simulink model "RemoteMicrogrid"  (R2025a)
settings: Solver=FixedStepAuto  StartTime=0.0  StopTime=8  FixedStep=Ts  MaxStep=1e-3  RelTol=1e-3
PreLoadFcn:
  | RemoteMicrogridInputData
undefined symbols (not defined in the file): BESS, ControlRoom, DiscIntNeverNeededParam, Grid, Load, Machine, Microgrid, MicrogridStatus, PV, relay1, T_on, Ts
libraries: ee_lib x53, fl_lib x39, eeGeneralControl x30, simulink x30, nesl_utility x26, nesl_utility_internal x19, slpidlib x7, eeTransforms x5, eeRmsMeasurement x4, eeTotalHarmonicDistorsion x4, batteryecm_lib x2, simulink_extras x2
(part 6 of 6)

== matlab function RemoteMicrogrid/Operator Control Room/Microgrid Control/Protection & Power Tracking/Overcurrent relay/Phase Protection Unit/Operating time /MATLAB Function ==
  data: plugSetting input; operatingTime output; timeSetting input; relayCharacteristic input
function operatingTime = fcn(plugSetting,timeSetting,relayCharacteristic)
   if plugSetting(1)>1 || plugSetting(2)>1 || plugSetting(3)>1  % Fault condition
    switch relayCharacteristic  % Selection of relay characteristic
        case 1                  % IEC Normal Inverse
          a=0.14;      
          b=0.02;
          c=0;
        case 2                  % IEC Very Inverse
           a=13.5;
           b=1;
           c=0;
        case 3                  % IEC Extremely Inverse
            a=80;
            b=2;
            c=0;
        case 4                  % IEC Moderately Inverse
            a=0.0515;
            b=0.02;
            c=0.114;
        case 5                  % IEEE Very Inverse
            a=19.61;
            b=2;
            c=0.491;
        case 6                  % IEEE Exteremely Inverse
            a=28.2;
            b=2;
            c=0.1217;
        otherwise               % Definite Time
            a=1;
            b=1;
            c=0;
            plugSetting=ones(3,1)*2;
    end           
         
         operatingTime=timeSetting*(a/(power(max(plugSetting),b)-1)+c);  % Calculate oeprating time of the relay  
   else
         operatingTime=inf;  % Set relay operating time to infinite if there is no fault
   end
end

== stateflow chart RemoteMicrogrid/Diesel Substation, BESS, & Microgrid Controller/Microgrid Controller/Microgrid Supervisory Control/Transition and Dispatch Control/On.Steady_State_Grid_Connected ==
  state Steady_State
    emergencyDispatch = false;
  state Resync_actions
    loadDispatch = true;
    LoadF2A = 0;
    LoadF2B = 0;
    loadReference = 0.1;
  (default) -> Steady_State
  Steady_State -> Resync_actions : after(0.2,sec)[resyncDispatch == true]
  data: LoadF2A output; LoadF2B output double; loadDispatch output boolean; loadReference output double; emergencyDispatch output boolean; resyncDispatch input boolean size=1

== stateflow chart RemoteMicrogrid/Diesel Substation, BESS, & Microgrid Controller/Microgrid Controller/Microgrid Supervisory Control/Transition and Dispatch Control/On.Resynchronization ==
  state Enable
    resync = true;
  state PCCBreakerClose
    resyncStatus = true;
    PCC = 0;
    resyncDispatch = true;
  (default) -> Enable
  Enable -> PCCBreakerClose : after(Resync.delay,sec)[Resync.status == true]
  data: Resync input Bus: Resync; PCC output double; resync output boolean; resyncDispatch output boolean size=1; resyncStatus output boolean

== stateflow chart RemoteMicrogrid/Diesel Substation, BESS, & Microgrid Controller/Microgrid Controller/Microgrid Supervisory Control/Transition and Dispatch Control/On.Steady_State_Islanded ==
  state Steady_state
    emergencyDispatch = false;
  state BreakerControl
    loadDispatch = true;
    LoadF2A = 1;
    LoadF2B = 1;
  (default) -> Steady_state
  Steady_state -> BreakerControl : after(0.5,sec)[plannedIslandingDispatch == true]
  data: LoadF2A output; LoadF2B output double; loadDispatch output boolean; plannedIslandingDispatch input boolean; emergencyDispatch output boolean

== stateflow chart RemoteMicrogrid/Diesel Substation, BESS, & Microgrid Controller/Microgrid Controller/Microgrid Supervisory Control/Transition and Dispatch Control/On.Unplanned_Islanding ==
  state TimeDelay
    loadDispatch = true;
    loadF2A = 1;
    loadF2B = 1;
    emergencyDispatch = true;
  state BreakerEnable
    PCC = 1;
  (default) -> TimeDelay
  TimeDelay -> BreakerEnable : after(0.05,sec)
  data: PCC output double; loadDispatch output boolean; loadF2A output double; loadF2B output double; emergencyDispatch output boolean
